simulink model "speedgoat_test_SN5659_R2021b_IO682"  (R2021b)
settings: Solver=FixedStepDiscrete  StartTime=0.0  StopTime=20  RelTol=1e-3
PreLoadFcn:
  | Ts_IO107 = 0.001;
  | Ts_IO107 = 0.001;
  | Ts_IO133 = 0.001
  | 
  | Ts_IO204 = 0.001;
  | 
  | 
  | Ts_IO503 = 0.01;
  | 
  | ts_IO612 = 1e-3;
  | Ts_IO682 = 0.005;
  | Ts_IO941 = 0.01;
InitFcn:
  | Ts_IO107 = 0.001;
  | Ts_IO107 = 0.001;
  | Ts_IO133 = 0.001
  | 
  | Ts_IO204 = 0.001;
  | 
  | 
  | Ts_IO503 = 0.01;
  | 
  | ts_IO612 = 1e-3;
  | Ts_IO682 = 0.005;
  | Ts_IO941 = 0.01;
StopFcn:
  | if isfile(['sdi_view_',bdroot,'.mldatx'])
  |  Simulink.sdi.clearPreferences();
  |  Simulink.sdi.view();
  |  pause(3);
  |  Simulink.sdi.loadView(['sdi_view_',bdroot,]);
  | end
undefined symbols (not defined in the file): IO682
libraries: speedgoatlib_IO682 x161, simulink x49
(part 1 of 3)
settings Model: Creator=yannick.orgas  LastModifiedBy=ACH
settings SolverCC: ConcurrentTasks=on  AlgebraicLoopSolver=TrustRegion  PositivePriorityOrder=on
settings DataIOCC: LimitDataPoints=on  SaveFormat=StructureWithTime
settings OptimizationCC: BlockReduction=off  OptimizeBlockIOStorage=off
settings DebuggingCC: TasksWithSamePriorityMsg=none  UnconnectedInputMsg=none  UnconnectedOutputMsg=none  UnconnectedLineMsg=none  SFMachineParentedDataDiag=warning
settings HardwareCC: ProdBitPerLong=64  ProdLongLongMode=on  ProdHWDeviceType=Intel->x86-64 (Linux 64)
settings RTWCC: Description=Simulink Real-Time  SystemTargetFile=slrealtime.tlc  TemplateMakefile=slrealtime_default_tmf  Toolchain=Simulink Real-Time Toolchain  BuildConfiguration=Faster Runs  CodeExecutionProfiling=on  TargetLang=C++
settings SimulinkRealTimeTargetCC: UseGCCFastMath=on

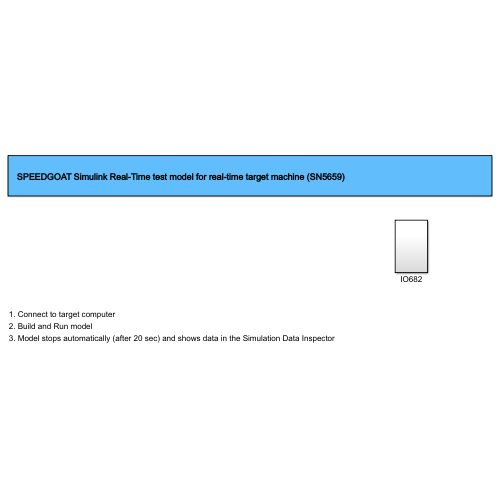
[thumbnail: Simulink's stored preview of the top-level diagram]
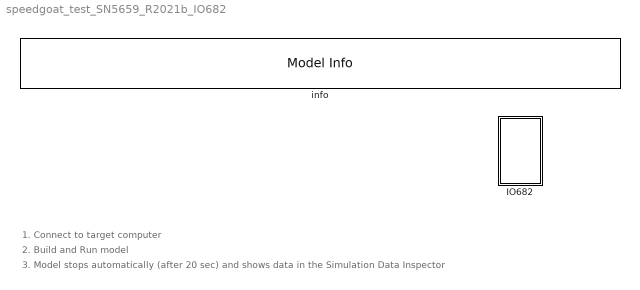
== system speedgoat_test_SN5659_R2021b_IO682 ==
  note: 1. Connect to target computer
  note: 2. Build and Run model
  note: 3. Model stops automatically (after 20 sec) and shows data in the Simulation Data Inspector
  IO682 : Subsystem
  info : simulink/Model-Wide Utilities/Model Info  Frame=on  DisplayStringWithTags=SPEEDGOAT Simulink Real-Time test model for real-time target machine (SN5659)  HorizontalTextAlignment=Left  LeftAlignmentValue=0.02

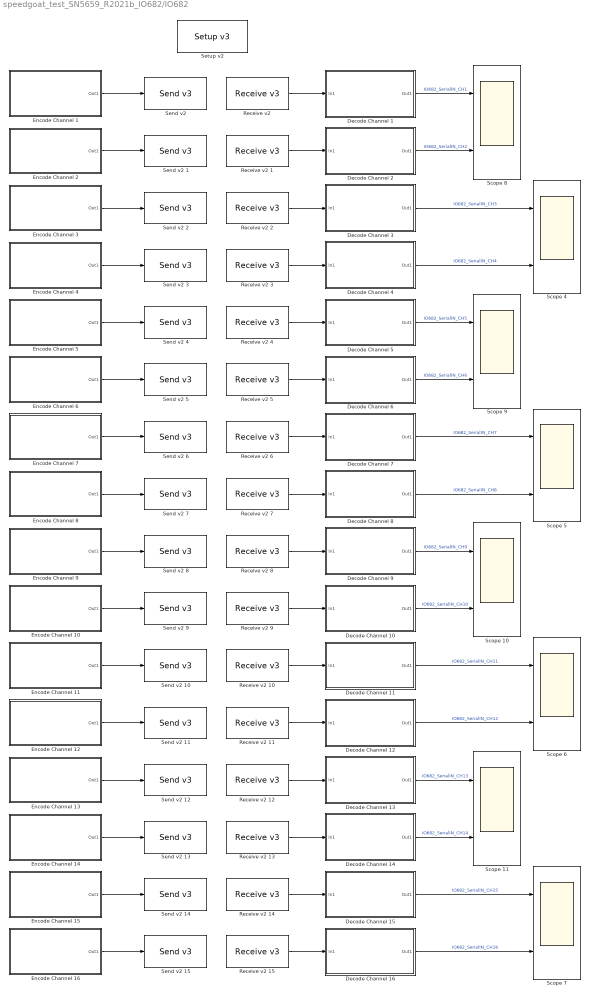
== system speedgoat_test_SN5659_R2021b_IO682/IO682 ==
  Decode Channel 1 : Subsystem
  Decode Channel 10 : Subsystem
  Decode Channel 11 : Subsystem
  Decode Channel 12 : Subsystem
  Decode Channel 13 : Subsystem
  Decode Channel 14 : Subsystem
  Decode Channel 15 : Subsystem
  Decode Channel 16 : Subsystem
  Decode Channel 2 : Subsystem
  Decode Channel 3 : Subsystem
  Decode Channel 4 : Subsystem
  Decode Channel 5 : Subsystem
  Decode Channel 6 : Subsystem
  Decode Channel 7 : Subsystem
  Decode Channel 8 : Subsystem
  Decode Channel 9 : Subsystem
  Encode Channel 1 : Subsystem
  Encode Channel 10 : Subsystem
  Encode Channel 11 : Subsystem
  Encode Channel 12 : Subsystem
  Encode Channel 13 : Subsystem
  Encode Channel 14 : Subsystem
  Encode Channel 15 : Subsystem
  Encode Channel 16 : Subsystem
  Encode Channel 2 : Subsystem
  Encode Channel 3 : Subsystem
  Encode Channel 4 : Subsystem
  Encode Channel 5 : Subsystem
  Encode Channel 6 : Subsystem
  Encode Channel 7 : Subsystem
  Encode Channel 8 : Subsystem
  Encode Channel 9 : Subsystem
  "Receive v2 " : speedgoatlib_IO682/Receive v3   parModuleId=1  parChannel=1  parMaxWords=50  parMinWords=1  parSampleTime=Ts_IO682
      settings: SourceProductName=Speedgoat I/O Blockset
  Receive v2 1 : speedgoatlib_IO682/Receive v3   parModuleId=1  parChannel=2  parMaxWords=50  parMinWords=1  parSampleTime=Ts_IO682
      settings: SourceProductName=Speedgoat I/O Blockset
  Receive v2 10 : speedgoatlib_IO682/Receive v3   parModuleId=1  parChannel=11  parMaxWords=50  parMinWords=1  parSampleTime=Ts_IO682
      settings: SourceProductName=Speedgoat I/O Blockset
  Receive v2 11 : speedgoatlib_IO682/Receive v3   parModuleId=1  parChannel=12  parMaxWords=50  parMinWords=1  parSampleTime=Ts_IO682
      settings: SourceProductName=Speedgoat I/O Blockset
  Receive v2 12 : speedgoatlib_IO682/Receive v3   parModuleId=1  parChannel=13  parMaxWords=50  parMinWords=1  parSampleTime=Ts_IO682
      settings: SourceProductName=Speedgoat I/O Blockset
  Receive v2 13 : speedgoatlib_IO682/Receive v3   parModuleId=1  parChannel=14  parMaxWords=50  parMinWords=1  parSampleTime=Ts_IO682
      settings: SourceProductName=Speedgoat I/O Blockset
  Receive v2 14 : speedgoatlib_IO682/Receive v3   parModuleId=1  parChannel=15  parMaxWords=50  parMinWords=1  parSampleTime=Ts_IO682
      settings: SourceProductName=Speedgoat I/O Blockset
  Receive v2 15 : speedgoatlib_IO682/Receive v3   parModuleId=1  parChannel=16  parMaxWords=50  parMinWords=1  parSampleTime=Ts_IO682
      settings: SourceProductName=Speedgoat I/O Blockset
  Receive v2 2 : speedgoatlib_IO682/Receive v3   parModuleId=1  parChannel=3  parMaxWords=50  parMinWords=1  parSampleTime=Ts_IO682
      settings: SourceProductName=Speedgoat I/O Blockset
  Receive v2 3 : speedgoatlib_IO682/Receive v3   parModuleId=1  parChannel=4  parMaxWords=50  parMinWords=1  parSampleTime=Ts_IO682
      settings: SourceProductName=Speedgoat I/O Blockset
  Receive v2 4 : speedgoatlib_IO682/Receive v3   parModuleId=1  parChannel=5  parMaxWords=50  parMinWords=1  parSampleTime=Ts_IO682
      settings: SourceProductName=Speedgoat I/O Blockset
  Receive v2 5 : speedgoatlib_IO682/Receive v3   parModuleId=1  parChannel=6  parMaxWords=50  parMinWords=1  parSampleTime=Ts_IO682
      settings: SourceProductName=Speedgoat I/O Blockset
  Receive v2 6 : speedgoatlib_IO682/Receive v3   parModuleId=1  parChannel=7  parMaxWords=50  parMinWords=1  parSampleTime=Ts_IO682
      settings: SourceProductName=Speedgoat I/O Blockset
  Receive v2 7 : speedgoatlib_IO682/Receive v3   parModuleId=1  parChannel=8  parMaxWords=50  parMinWords=1  parSampleTime=Ts_IO682
      settings: SourceProductName=Speedgoat I/O Blockset
  Receive v2 8 : speedgoatlib_IO682/Receive v3   parModuleId=1  parChannel=9  parMaxWords=50  parMinWords=1  parSampleTime=Ts_IO682
      settings: SourceProductName=Speedgoat I/O Blockset
  Receive v2 9 : speedgoatlib_IO682/Receive v3   parModuleId=1  parChannel=10  parMaxWords=50  parMinWords=1  parSampleTime=Ts_IO682
      settings: SourceProductName=Speedgoat I/O Blockset
  Scope {4..11} (8 alike) : Scope  NumInputPorts=2
  "Send v2 " : speedgoatlib_IO682/Send v3   parModuleId=1  parChannel=1  parSampleTime=Ts_IO682
      settings: SourceProductName=Speedgoat I/O Blockset
  Send v2 1 : speedgoatlib_IO682/Send v3   parModuleId=1  parChannel=2  parSampleTime=Ts_IO682
      settings: SourceProductName=Speedgoat I/O Blockset
  Send v2 10 : speedgoatlib_IO682/Send v3   parModuleId=1  parChannel=11  parSampleTime=Ts_IO682
      settings: SourceProductName=Speedgoat I/O Blockset
  Send v2 11 : speedgoatlib_IO682/Send v3   parModuleId=1  parChannel=12  parSampleTime=Ts_IO682
      settings: SourceProductName=Speedgoat I/O Blockset
  Send v2 12 : speedgoatlib_IO682/Send v3   parModuleId=1  parChannel=13  parSampleTime=Ts_IO682
      settings: SourceProductName=Speedgoat I/O Blockset
  Send v2 13 : speedgoatlib_IO682/Send v3   parModuleId=1  parChannel=14  parSampleTime=Ts_IO682
      settings: SourceProductName=Speedgoat I/O Blockset
  Send v2 14 : speedgoatlib_IO682/Send v3   parModuleId=1  parChannel=15  parSampleTime=Ts_IO682
      settings: SourceProductName=Speedgoat I/O Blockset
  Send v2 15 : speedgoatlib_IO682/Send v3   parModuleId=1  parChannel=16  parSampleTime=Ts_IO682
      settings: SourceProductName=Speedgoat I/O Blockset
  Send v2 2 : speedgoatlib_IO682/Send v3   parModuleId=1  parChannel=3  parSampleTime=Ts_IO682
      settings: SourceProductName=Speedgoat I/O Blockset
  Send v2 3 : speedgoatlib_IO682/Send v3   parModuleId=1  parChannel=4  parSampleTime=Ts_IO682
      settings: SourceProductName=Speedgoat I/O Blockset
  Send v2 4 : speedgoatlib_IO682/Send v3   parModuleId=1  parChannel=5  parSampleTime=Ts_IO682
      settings: SourceProductName=Speedgoat I/O Blockset
  Send v2 5 : speedgoatlib_IO682/Send v3   parModuleId=1  parChannel=6  parSampleTime=Ts_IO682
      settings: SourceProductName=Speedgoat I/O Blockset
  Send v2 6 : speedgoatlib_IO682/Send v3   parModuleId=1  parChannel=7  parSampleTime=Ts_IO682
      settings: SourceProductName=Speedgoat I/O Blockset
  Send v2 7 : speedgoatlib_IO682/Send v3   parModuleId=1  parChannel=8  parSampleTime=Ts_IO682
      settings: SourceProductName=Speedgoat I/O Blockset
  Send v2 8 : speedgoatlib_IO682/Send v3   parModuleId=1  parChannel=9  parSampleTime=Ts_IO682
      settings: SourceProductName=Speedgoat I/O Blockset
  Send v2 9 : speedgoatlib_IO682/Send v3   parModuleId=1  parChannel=10  parSampleTime=Ts_IO682
      settings: SourceProductName=Speedgoat I/O Blockset
  "Setup v2 " : speedgoatlib_IO682/Setup v3   parModuleId=1  parBoardVariant=IO682-16-16  parPciSlot=-1  parTimerCount=4000  parChannelMode=Manual  parInBitRate1=100000  parInBufferMode1=Individual  parInEnable1=on  parInParity1=on  parInInternalWrap1=off  parInBitRate2=100000  parInBufferMode2=Individual  parInEnable2=on  parInParity2=on  parInInternalWrap2=off  parInBitRate3=100000  parInBufferMode3=Individual  parInEnable3=on  parInParity3=on  parInInternalWrap3=off  parInBitRate4=100000  parInBufferMode4=Individual  parInEnable4=on  parInParity4=on  parInInternalWrap4=off  parInBitRate5=100000  parInBufferMode5=Individual  parInEnable5=on  parInParity5=on  parInInternalWrap5=off  parInBitRate6=100000  parInBufferMode6=Individual  parInEnable6=on  parInParity6=on  parInInternalWrap6=off  parInBitRate7=100000  parInBufferMode7=Individual  parInEnable7=on  parInParity7=on  parInInternalWrap7=off  parInBitRate8=100000  parInBufferMode8=Individual  parInEnable8=on  parInParity8=on  parInInternalWrap8=off  parInBitRate9=100000  parInBufferMode9=Individual  parInEnable9=on  parInParity9=on  parInInternalWrap9=off  parInBitRate10=100000  parInBufferMode10=Individual  parInEnable10=on  parInParity10=on  parInInternalWrap10=off  parInBitRate11=100000  parInBufferMode11=Individual  parInEnable11=on  parInParity11=on  parInInternalWrap11=off  parInBitRate12=100000  parInBufferMode12=Individual  parInEnable12=on  parInParity12=on  parInInternalWrap12=off  parInBitRate13=100000  parInBufferMode13=Individual  parInEnable13=on  parInParity13=on  parInInternalWrap13=off  parInBitRate14=100000  parInBufferMode14=Individual  parInEnable14=on  parInParity14=on  parInInternalWrap14=off  parInBitRate15=100000  parInBufferMode15=Individual  parInEnable15=on  parInParity15=on  parInInternalWrap15=off  parInBitRate16=100000  parInBufferMode16=Individual  parInEnable16=on  parInParity16=on  parInInternalWrap16=off  parOutBitRate1=100000  parOutParity1=Odd  parOutProtocolError1=None  parOutEnable1=on  parOutBitRate2=100000  parOutParity2=Odd  parOutProtocolError2=None  parOutEnable2=on  parOutBitRate3=100000  parOutParity3=Odd  parOutProtocolError3=None  parOutEnable3=on  parOutBitRate4=100000  parOutParity4=Odd  parOutProtocolError4=None  parOutEnable4=on  parOutBitRate5=100000  parOutParity5=Odd  parOutProtocolError5=None  parOutEnable5=on  parOutBitRate6=100000  parOutParity6=Odd  parOutProtocolError6=None  parOutEnable6=on  parOutBitRate7=100000  parOutParity7=Odd  parOutProtocolError7=None  parOutEnable7=on  parOutBitRate8=100000  parOutParity8=Odd  parOutProtocolError8=None  parOutEnable8=on  parOutBitRate9=100000  parOutParity9=Odd  parOutProtocolError9=None  parOutEnable9=on  parOutBitRate10=100000  parOutParity10=Odd  parOutProtocolError10=None  parOutEnable10=on  parOutBitRate11=100000  parOutParity11=Odd  parOutProtocolError11=None  parOutEnable11=on  parOutBitRate12=100000  parOutParity12=Odd  parOutProtocolError12=None  parOutEnable12=on  parOutBitRate13=100000  parOutParity13=Odd  parOutProtocolError13=None  parOutEnable13=on  parOutBitRate14=100000  parOutParity14=Odd  parOutProtocolError14=None  parOutEnable14=on  parOutBitRate15=100000  parOutParity15=Odd  parOutProtocolError15=None  parOutEnable15=on  parOutBitRate16=100000  parOutParity16=Odd  parOutProtocolError16=None  parOutEnable16=on  parChConfigFile=''  parScheduleMode=Manual  parScheduledMsgConfigFile=''  parHwDeviceId=hex2dec('0830')  parTimeSource=Internal timer  parChInConfig=[158 8 7 7 1;158 8 7 7 1;158 8 7 7 1;158 8 7 7 1;158 8 7 7 1;158 8 7 7 1;158 8 7 7 1;158 8 7 7 1;158 8 7 7 1;158 8 7 7 1;158 8 7 7 1;158 8 7 7 1;158 8 7 7 1;158 8 7 7 1;158 8 7 7 1;158 8 7 7 1]  parChOutConfig=[158 0 4 7;158 0 4 7;158 0 4 7;158 0 4 7;158 0 4 7;158 0 4 7;158 0 4 7;158 0 4 7;158 0 4 7;158 0 4 7;158 0 4 7;158 0 4 7;158 0 4 7;158 0 4 7;158 0 4 7;158 0 4 7]  parScheduledMessages=0
      settings: SourceProductName=Speedgoat I/O Blockset
  wires:
  Receive v2 3/1 -> Decode Channel 4/1(In1)
  Decode Channel 15/1(Out1) -> Scope 7/1  "IO682_SerialIN_CH15"
  "Receive v2 "/1 -> Decode Channel 1/1(In1)
  Receive v2 13/1 -> Decode Channel 14/1(In1)
  Decode Channel 11/1(Out1) -> Scope 6/1  "IO682_SerialIN_CH11"
  Encode Channel 15/1(Out1) -> Send v2 14/1
  Receive v2 8/1 -> Decode Channel 9/1(In1)
  Decode Channel 16/1(Out1) -> Scope 7/2  "IO682_SerialIN_CH16"
  Receive v2 15/1 -> Decode Channel 16/1(In1)
  Encode Channel 13/1(Out1) -> Send v2 12/1
  Encode Channel 14/1(Out1) -> Send v2 13/1
  Decode Channel 12/1(Out1) -> Scope 6/2  "IO682_SerialIN_CH12"
  Decode Channel 3/1(Out1) -> Scope 4/1  "IO682_SerialIN_CH3"
  Receive v2 14/1 -> Decode Channel 15/1(In1)
  Encode Channel 1/1(Out1) -> "Send v2 "/1
  Decode Channel 5/1(Out1) -> Scope 9/1  "IO682_SerialIN_CH5"
  Encode Channel 7/1(Out1) -> Send v2 6/1
  Receive v2 7/1 -> Decode Channel 8/1(In1)
  Decode Channel 14/1(Out1) -> Scope 11/2  "IO682_SerialIN_CH14"
  Decode Channel 10/1(Out1) -> Scope 10/2  "IO682_SerialIN_CH10"
  Encode Channel 9/1(Out1) -> Send v2 8/1
  Receive v2 2/1 -> Decode Channel 3/1(In1)
  Receive v2 10/1 -> Decode Channel 11/1(In1)
  Decode Channel 8/1(Out1) -> Scope 5/2  "IO682_SerialIN_CH8"
  Encode Channel 4/1(Out1) -> Send v2 3/1
  Encode Channel 6/1(Out1) -> Send v2 5/1
  Encode Channel 2/1(Out1) -> Send v2 1/1
  Receive v2 9/1 -> Decode Channel 10/1(In1)
  Encode Channel 16/1(Out1) -> Send v2 15/1
  Decode Channel 9/1(Out1) -> Scope 10/1  "IO682_SerialIN_CH9"
  Receive v2 11/1 -> Decode Channel 12/1(In1)
  Encode Channel 11/1(Out1) -> Send v2 10/1
  Encode Channel 10/1(Out1) -> Send v2 9/1
  Receive v2 12/1 -> Decode Channel 13/1(In1)
  Decode Channel 1/1(Out1) -> Scope 8/1  "IO682_SerialIN_CH1"
  Decode Channel 2/1(Out1) -> Scope 8/2  "IO682_SerialIN_CH2"
  Decode Channel 13/1(Out1) -> Scope 11/1  "IO682_SerialIN_CH13"
  Decode Channel 6/1(Out1) -> Scope 9/2  "IO682_SerialIN_CH6"
  Receive v2 1/1 -> Decode Channel 2/1(In1)
  Encode Channel 8/1(Out1) -> Send v2 7/1
  Receive v2 5/1 -> Decode Channel 6/1(In1)
  Receive v2 4/1 -> Decode Channel 5/1(In1)
  Decode Channel 7/1(Out1) -> Scope 5/1  "IO682_SerialIN_CH7"
  Encode Channel 5/1(Out1) -> Send v2 4/1
  Receive v2 6/1 -> Decode Channel 7/1(In1)
  Decode Channel 4/1(Out1) -> Scope 4/2  "IO682_SerialIN_CH4"
  Encode Channel 3/1(Out1) -> Send v2 2/1
  Encode Channel 12/1(Out1) -> Send v2 11/1

== system speedgoat_test_SN5659_R2021b_IO682/IO682/Decode Channel 1 ==
  note: Because of the limited number of bits
      | that are encoded and sent by ARINC,
      | these values may differ from values
      | on the input side.
  In1 : Inport
  Decode 1 : speedgoatlib_IO682/Decode v2   parMode=Standard  parLabel=100  parDataType=[1]  parResolution=[1024]  parSyncMask=hex2dec('0x0')  parSyncValue=hex2dec('0x0')  parCustomDataType=Raw  parDataLSB=9  parDataMSB=31  parBitPosition=[9, 31]  parScaleBNR=1  parExponent=8  parMantissa=14  parTimeTags=off  parHoldLastVal=on  parStatus=off
      settings: SourceProductName=Simulink Real-Time: Speedgoat I/O Blockset
  Decode 3 : speedgoatlib_IO682/Decode v2   parMode=Standard  parLabel=102  parDataType=[1]  parResolution=[65536]  parSyncMask=hex2dec('0x0')  parSyncValue=hex2dec('0x0')  parCustomDataType=Raw  parDataLSB=9  parDataMSB=31  parBitPosition=[9, 31]  parScaleBNR=1  parExponent=8  parMantissa=14  parTimeTags=off  parHoldLastVal=on  parStatus=off
      settings: SourceProductName=Simulink Real-Time: Speedgoat I/O Blockset
  Decode 4 : speedgoatlib_IO682/Decode v2   parMode=Standard  parLabel=103  parDataType=[1]  parResolution=[1024]  parSyncMask=hex2dec('0x0')  parSyncValue=hex2dec('0x0')  parCustomDataType=Raw  parDataLSB=9  parDataMSB=31  parBitPosition=[9, 31]  parScaleBNR=1  parExponent=8  parMantissa=14  parTimeTags=off  parHoldLastVal=on  parStatus=off
      settings: SourceProductName=Simulink Real-Time: Speedgoat I/O Blockset
  Decode 5 : speedgoatlib_IO682/Decode v2   parMode=Standard  parLabel=101  parDataType=[2]  parResolution=[.1]  parSyncMask=hex2dec('0x0')  parSyncValue=hex2dec('0x0')  parCustomDataType=Raw  parDataLSB=9  parDataMSB=31  parBitPosition=[9, 31]  parScaleBNR=1  parExponent=8  parMantissa=14  parTimeTags=off  parHoldLastVal=on  parStatus=off
      settings: SourceProductName=Simulink Real-Time: Speedgoat I/O Blockset
  Mux : Mux
  Out1 : Outport
  wires:
  In1/1 -> Decode 3/1, Decode 4/1, Decode 5/1, Decode 1/1
  Mux/1 -> Out1/1
  Decode 5/1 -> Mux/2
  Decode 1/1 -> Mux/1
  Decode 3/1 -> Mux/3
  Decode 4/1 -> Mux/4

== system speedgoat_test_SN5659_R2021b_IO682/IO682/Decode Channel 10 ==
  In1 : Inport
  Decode 1 : speedgoatlib_IO682/Decode v2   parMode=Standard  parLabel=100  parDataType=[1]  parResolution=[1024]  parSyncMask=hex2dec('0x0')  parSyncValue=hex2dec('0x0')  parCustomDataType=Raw  parDataLSB=9  parDataMSB=31  parBitPosition=[9, 31]  parScaleBNR=1  parExponent=8  parMantissa=14  parTimeTags=off  parHoldLastVal=on  parStatus=off
      settings: SourceProductName=Simulink Real-Time: Speedgoat I/O Blockset
  Decode 2 : speedgoatlib_IO682/Decode v2   parMode=Standard  parLabel=101  parDataType=[2]  parResolution=[.1]  parSyncMask=hex2dec('0x0')  parSyncValue=hex2dec('0x0')  parCustomDataType=Raw  parDataLSB=9  parDataMSB=31  parBitPosition=[9, 31]  parScaleBNR=1  parExponent=8  parMantissa=14  parTimeTags=off  parHoldLastVal=on  parStatus=off
      settings: SourceProductName=Simulink Real-Time: Speedgoat I/O Blockset
  Decode 3 : speedgoatlib_IO682/Decode v2   parMode=Standard  parLabel=102  parDataType=[1]  parResolution=[65536]  parSyncMask=hex2dec('0x0')  parSyncValue=hex2dec('0x0')  parCustomDataType=Raw  parDataLSB=9  parDataMSB=31  parBitPosition=[9, 31]  parScaleBNR=1  parExponent=8  parMantissa=14  parTimeTags=off  parHoldLastVal=on  parStatus=off
      settings: SourceProductName=Simulink Real-Time: Speedgoat I/O Blockset
  Decode 4 : speedgoatlib_IO682/Decode v2   parMode=Standard  parLabel=103  parDataType=[1]  parResolution=[1024]  parSyncMask=hex2dec('0x0')  parSyncValue=hex2dec('0x0')  parCustomDataType=Raw  parDataLSB=9  parDataMSB=31  parBitPosition=[9, 31]  parScaleBNR=1  parExponent=8  parMantissa=14  parTimeTags=off  parHoldLastVal=on  parStatus=off
      settings: SourceProductName=Simulink Real-Time: Speedgoat I/O Blockset
  Mux : Mux
  Out1 : Outport
  wires:
  Decode 1/1 -> Mux/1
  In1/1 -> Decode 4/1, Decode 3/1, Decode 2/1, Decode 1/1
  Mux/1 -> Out1/1
  Decode 4/1 -> Mux/4
  Decode 3/1 -> Mux/3
  Decode 2/1 -> Mux/2

== system speedgoat_test_SN5659_R2021b_IO682/IO682/Decode Channel 11 ==
  In1 : Inport
  Decode 1 : speedgoatlib_IO682/Decode v2   parMode=Standard  parLabel=100  parDataType=[1]  parResolution=[1024]  parSyncMask=hex2dec('0x0')  parSyncValue=hex2dec('0x0')  parCustomDataType=Raw  parDataLSB=9  parDataMSB=31  parBitPosition=[9, 31]  parScaleBNR=1  parExponent=8  parMantissa=14  parTimeTags=off  parHoldLastVal=on  parStatus=off
      settings: SourceProductName=Simulink Real-Time: Speedgoat I/O Blockset
  Decode 2 : speedgoatlib_IO682/Decode v2   parMode=Standard  parLabel=101  parDataType=[2]  parResolution=[.1]  parSyncMask=hex2dec('0x0')  parSyncValue=hex2dec('0x0')  parCustomDataType=Raw  parDataLSB=9  parDataMSB=31  parBitPosition=[9, 31]  parScaleBNR=1  parExponent=8  parMantissa=14  parTimeTags=off  parHoldLastVal=on  parStatus=off
      settings: SourceProductName=Simulink Real-Time: Speedgoat I/O Blockset
  Decode 3 : speedgoatlib_IO682/Decode v2   parMode=Standard  parLabel=102  parDataType=[1]  parResolution=[65536]  parSyncMask=hex2dec('0x0')  parSyncValue=hex2dec('0x0')  parCustomDataType=Raw  parDataLSB=9  parDataMSB=31  parBitPosition=[9, 31]  parScaleBNR=1  parExponent=8  parMantissa=14  parTimeTags=off  parHoldLastVal=on  parStatus=off
      settings: SourceProductName=Simulink Real-Time: Speedgoat I/O Blockset
  Decode 4 : speedgoatlib_IO682/Decode v2   parMode=Standard  parLabel=103  parDataType=[1]  parResolution=[1024]  parSyncMask=hex2dec('0x0')  parSyncValue=hex2dec('0x0')  parCustomDataType=Raw  parDataLSB=9  parDataMSB=31  parBitPosition=[9, 31]  parScaleBNR=1  parExponent=8  parMantissa=14  parTimeTags=off  parHoldLastVal=on  parStatus=off
      settings: SourceProductName=Simulink Real-Time: Speedgoat I/O Blockset
  Mux : Mux
  Out1 : Outport
  wires:
  Decode 1/1 -> Mux/1
  Decode 2/1 -> Mux/2
  Decode 4/1 -> Mux/4
  Decode 3/1 -> Mux/3
  Mux/1 -> Out1/1
  In1/1 -> Decode 4/1, Decode 3/1, Decode 2/1, Decode 1/1

== system speedgoat_test_SN5659_R2021b_IO682/IO682/Decode Channel 12 ==
  In1 : Inport
  Decode 1 : speedgoatlib_IO682/Decode v2   parMode=Standard  parLabel=100  parDataType=[1]  parResolution=[1024]  parSyncMask=hex2dec('0x0')  parSyncValue=hex2dec('0x0')  parCustomDataType=Raw  parDataLSB=9  parDataMSB=31  parBitPosition=[9, 31]  parScaleBNR=1  parExponent=8  parMantissa=14  parTimeTags=off  parHoldLastVal=on  parStatus=off
      settings: SourceProductName=Simulink Real-Time: Speedgoat I/O Blockset
  Decode 2 : speedgoatlib_IO682/Decode v2   parMode=Standard  parLabel=101  parDataType=[2]  parResolution=[.1]  parSyncMask=hex2dec('0x0')  parSyncValue=hex2dec('0x0')  parCustomDataType=Raw  parDataLSB=9  parDataMSB=31  parBitPosition=[9, 31]  parScaleBNR=1  parExponent=8  parMantissa=14  parTimeTags=off  parHoldLastVal=on  parStatus=off
      settings: SourceProductName=Simulink Real-Time: Speedgoat I/O Blockset
  Decode 3 : speedgoatlib_IO682/Decode v2   parMode=Standard  parLabel=102  parDataType=[1]  parResolution=[65536]  parSyncMask=hex2dec('0x0')  parSyncValue=hex2dec('0x0')  parCustomDataType=Raw  parDataLSB=9  parDataMSB=31  parBitPosition=[9, 31]  parScaleBNR=1  parExponent=8  parMantissa=14  parTimeTags=off  parHoldLastVal=on  parStatus=off
      settings: SourceProductName=Simulink Real-Time: Speedgoat I/O Blockset
  Decode 4 : speedgoatlib_IO682/Decode v2   parMode=Standard  parLabel=103  parDataType=[1]  parResolution=[1024]  parSyncMask=hex2dec('0x0')  parSyncValue=hex2dec('0x0')  parCustomDataType=Raw  parDataLSB=9  parDataMSB=31  parBitPosition=[9, 31]  parScaleBNR=1  parExponent=8  parMantissa=14  parTimeTags=off  parHoldLastVal=on  parStatus=off
      settings: SourceProductName=Simulink Real-Time: Speedgoat I/O Blockset
  Mux : Mux
  Out1 : Outport
  wires:
  Decode 1/1 -> Mux/1
  Decode 2/1 -> Mux/2
  Decode 4/1 -> Mux/4
  Decode 3/1 -> Mux/3
  Mux/1 -> Out1/1
  In1/1 -> Decode 4/1, Decode 3/1, Decode 2/1, Decode 1/1

== system speedgoat_test_SN5659_R2021b_IO682/IO682/Decode Channel 13 ==
  note: Because of the limited number of bits
      | that are encoded and sent by ARINC,
      | these values may differ from values
      | on the input side.
  In1 : Inport
  Decode 1 : speedgoatlib_IO682/Decode v2   parMode=Standard  parLabel=100  parDataType=[1]  parResolution=[1024]  parSyncMask=hex2dec('0x0')  parSyncValue=hex2dec('0x0')  parCustomDataType=Raw  parDataLSB=9  parDataMSB=31  parBitPosition=[9, 31]  parScaleBNR=1  parExponent=8  parMantissa=14  parTimeTags=off  parHoldLastVal=on  parStatus=off
      settings: SourceProductName=Simulink Real-Time: Speedgoat I/O Blockset
  Decode 3 : speedgoatlib_IO682/Decode v2   parMode=Standard  parLabel=102  parDataType=[1]  parResolution=[65536]  parSyncMask=hex2dec('0x0')  parSyncValue=hex2dec('0x0')  parCustomDataType=Raw  parDataLSB=9  parDataMSB=31  parBitPosition=[9, 31]  parScaleBNR=1  parExponent=8  parMantissa=14  parTimeTags=off  parHoldLastVal=on  parStatus=off
      settings: SourceProductName=Simulink Real-Time: Speedgoat I/O Blockset
  Decode 4 : speedgoatlib_IO682/Decode v2   parMode=Standard  parLabel=103  parDataType=[1]  parResolution=[1024]  parSyncMask=hex2dec('0x0')  parSyncValue=hex2dec('0x0')  parCustomDataType=Raw  parDataLSB=9  parDataMSB=31  parBitPosition=[9, 31]  parScaleBNR=1  parExponent=8  parMantissa=14  parTimeTags=off  parHoldLastVal=on  parStatus=off
      settings: SourceProductName=Simulink Real-Time: Speedgoat I/O Blockset
  Decode 5 : speedgoatlib_IO682/Decode v2   parMode=Standard  parLabel=101  parDataType=[2]  parResolution=[.1]  parSyncMask=hex2dec('0x0')  parSyncValue=hex2dec('0x0')  parCustomDataType=Raw  parDataLSB=9  parDataMSB=31  parBitPosition=[9, 31]  parScaleBNR=1  parExponent=8  parMantissa=14  parTimeTags=off  parHoldLastVal=on  parStatus=off
      settings: SourceProductName=Simulink Real-Time: Speedgoat I/O Blockset
  Mux : Mux
  Out1 : Outport
  wires:
  In1/1 -> Decode 3/1, Decode 4/1, Decode 5/1, Decode 1/1
  Mux/1 -> Out1/1
  Decode 5/1 -> Mux/2
  Decode 1/1 -> Mux/1
  Decode 3/1 -> Mux/3
  Decode 4/1 -> Mux/4

== system speedgoat_test_SN5659_R2021b_IO682/IO682/Decode Channel 14 ==
  In1 : Inport
  Decode 1 : speedgoatlib_IO682/Decode v2   parMode=Standard  parLabel=100  parDataType=[1]  parResolution=[1024]  parSyncMask=hex2dec('0x0')  parSyncValue=hex2dec('0x0')  parCustomDataType=Raw  parDataLSB=9  parDataMSB=31  parBitPosition=[9, 31]  parScaleBNR=1  parExponent=8  parMantissa=14  parTimeTags=off  parHoldLastVal=on  parStatus=off
      settings: SourceProductName=Simulink Real-Time: Speedgoat I/O Blockset
  Decode 2 : speedgoatlib_IO682/Decode v2   parMode=Standard  parLabel=101  parDataType=[2]  parResolution=[.1]  parSyncMask=hex2dec('0x0')  parSyncValue=hex2dec('0x0')  parCustomDataType=Raw  parDataLSB=9  parDataMSB=31  parBitPosition=[9, 31]  parScaleBNR=1  parExponent=8  parMantissa=14  parTimeTags=off  parHoldLastVal=on  parStatus=off
      settings: SourceProductName=Simulink Real-Time: Speedgoat I/O Blockset
  Decode 3 : speedgoatlib_IO682/Decode v2   parMode=Standard  parLabel=102  parDataType=[1]  parResolution=[65536]  parSyncMask=hex2dec('0x0')  parSyncValue=hex2dec('0x0')  parCustomDataType=Raw  parDataLSB=9  parDataMSB=31  parBitPosition=[9, 31]  parScaleBNR=1  parExponent=8  parMantissa=14  parTimeTags=off  parHoldLastVal=on  parStatus=off
      settings: SourceProductName=Simulink Real-Time: Speedgoat I/O Blockset
  Decode 4 : speedgoatlib_IO682/Decode v2   parMode=Standard  parLabel=103  parDataType=[1]  parResolution=[1024]  parSyncMask=hex2dec('0x0')  parSyncValue=hex2dec('0x0')  parCustomDataType=Raw  parDataLSB=9  parDataMSB=31  parBitPosition=[9, 31]  parScaleBNR=1  parExponent=8  parMantissa=14  parTimeTags=off  parHoldLastVal=on  parStatus=off
      settings: SourceProductName=Simulink Real-Time: Speedgoat I/O Blockset
  Mux : Mux
  Out1 : Outport
  wires:
  Decode 1/1 -> Mux/1
  In1/1 -> Decode 4/1, Decode 3/1, Decode 2/1, Decode 1/1
  Mux/1 -> Out1/1
  Decode 4/1 -> Mux/4
  Decode 3/1 -> Mux/3
  Decode 2/1 -> Mux/2

== system speedgoat_test_SN5659_R2021b_IO682/IO682/Decode Channel 15 ==
  In1 : Inport
  Decode 1 : speedgoatlib_IO682/Decode v2   parMode=Standard  parLabel=100  parDataType=[1]  parResolution=[1024]  parSyncMask=hex2dec('0x0')  parSyncValue=hex2dec('0x0')  parCustomDataType=Raw  parDataLSB=9  parDataMSB=31  parBitPosition=[9, 31]  parScaleBNR=1  parExponent=8  parMantissa=14  parTimeTags=off  parHoldLastVal=on  parStatus=off
      settings: SourceProductName=Simulink Real-Time: Speedgoat I/O Blockset
  Decode 2 : speedgoatlib_IO682/Decode v2   parMode=Standard  parLabel=101  parDataType=[2]  parResolution=[.1]  parSyncMask=hex2dec('0x0')  parSyncValue=hex2dec('0x0')  parCustomDataType=Raw  parDataLSB=9  parDataMSB=31  parBitPosition=[9, 31]  parScaleBNR=1  parExponent=8  parMantissa=14  parTimeTags=off  parHoldLastVal=on  parStatus=off
      settings: SourceProductName=Simulink Real-Time: Speedgoat I/O Blockset
  Decode 3 : speedgoatlib_IO682/Decode v2   parMode=Standard  parLabel=102  parDataType=[1]  parResolution=[65536]  parSyncMask=hex2dec('0x0')  parSyncValue=hex2dec('0x0')  parCustomDataType=Raw  parDataLSB=9  parDataMSB=31  parBitPosition=[9, 31]  parScaleBNR=1  parExponent=8  parMantissa=14  parTimeTags=off  parHoldLastVal=on  parStatus=off
      settings: SourceProductName=Simulink Real-Time: Speedgoat I/O Blockset
  Decode 4 : speedgoatlib_IO682/Decode v2   parMode=Standard  parLabel=103  parDataType=[1]  parResolution=[1024]  parSyncMask=hex2dec('0x0')  parSyncValue=hex2dec('0x0')  parCustomDataType=Raw  parDataLSB=9  parDataMSB=31  parBitPosition=[9, 31]  parScaleBNR=1  parExponent=8  parMantissa=14  parTimeTags=off  parHoldLastVal=on  parStatus=off
      settings: SourceProductName=Simulink Real-Time: Speedgoat I/O Blockset
  Mux : Mux
  Out1 : Outport
  wires:
  Decode 1/1 -> Mux/1
  Decode 2/1 -> Mux/2
  Decode 4/1 -> Mux/4
  Decode 3/1 -> Mux/3
  Mux/1 -> Out1/1
  In1/1 -> Decode 4/1, Decode 3/1, Decode 2/1, Decode 1/1

== system speedgoat_test_SN5659_R2021b_IO682/IO682/Decode Channel 16 ==
  In1 : Inport
  Decode 1 : speedgoatlib_IO682/Decode v2   parMode=Standard  parLabel=100  parDataType=[1]  parResolution=[1024]  parSyncMask=hex2dec('0x0')  parSyncValue=hex2dec('0x0')  parCustomDataType=Raw  parDataLSB=9  parDataMSB=31  parBitPosition=[9, 31]  parScaleBNR=1  parExponent=8  parMantissa=14  parTimeTags=off  parHoldLastVal=on  parStatus=off
      settings: SourceProductName=Simulink Real-Time: Speedgoat I/O Blockset
  Decode 2 : speedgoatlib_IO682/Decode v2   parMode=Standard  parLabel=101  parDataType=[2]  parResolution=[.1]  parSyncMask=hex2dec('0x0')  parSyncValue=hex2dec('0x0')  parCustomDataType=Raw  parDataLSB=9  parDataMSB=31  parBitPosition=[9, 31]  parScaleBNR=1  parExponent=8  parMantissa=14  parTimeTags=off  parHoldLastVal=on  parStatus=off
      settings: SourceProductName=Simulink Real-Time: Speedgoat I/O Blockset
  Decode 3 : speedgoatlib_IO682/Decode v2   parMode=Standard  parLabel=102  parDataType=[1]  parResolution=[65536]  parSyncMask=hex2dec('0x0')  parSyncValue=hex2dec('0x0')  parCustomDataType=Raw  parDataLSB=9  parDataMSB=31  parBitPosition=[9, 31]  parScaleBNR=1  parExponent=8  parMantissa=14  parTimeTags=off  parHoldLastVal=on  parStatus=off
      settings: SourceProductName=Simulink Real-Time: Speedgoat I/O Blockset
  Decode 4 : speedgoatlib_IO682/Decode v2   parMode=Standard  parLabel=103  parDataType=[1]  parResolution=[1024]  parSyncMask=hex2dec('0x0')  parSyncValue=hex2dec('0x0')  parCustomDataType=Raw  parDataLSB=9  parDataMSB=31  parBitPosition=[9, 31]  parScaleBNR=1  parExponent=8  parMantissa=14  parTimeTags=off  parHoldLastVal=on  parStatus=off
      settings: SourceProductName=Simulink Real-Time: Speedgoat I/O Blockset
  Mux : Mux
  Out1 : Outport
  wires:
  Decode 1/1 -> Mux/1
  Decode 2/1 -> Mux/2
  Decode 4/1 -> Mux/4
  Decode 3/1 -> Mux/3
  Mux/1 -> Out1/1
  In1/1 -> Decode 4/1, Decode 3/1, Decode 2/1, Decode 1/1

== system speedgoat_test_SN5659_R2021b_IO682/IO682/Decode Channel 2 ==
  In1 : Inport
  Decode 1 : speedgoatlib_IO682/Decode v2   parMode=Standard  parLabel=100  parDataType=[1]  parResolution=[1024]  parSyncMask=hex2dec('0x0')  parSyncValue=hex2dec('0x0')  parCustomDataType=Raw  parDataLSB=9  parDataMSB=31  parBitPosition=[9, 31]  parScaleBNR=1  parExponent=8  parMantissa=14  parTimeTags=off  parHoldLastVal=on  parStatus=off
      settings: SourceProductName=Simulink Real-Time: Speedgoat I/O Blockset
  Decode 2 : speedgoatlib_IO682/Decode v2   parMode=Standard  parLabel=101  parDataType=[2]  parResolution=[.1]  parSyncMask=hex2dec('0x0')  parSyncValue=hex2dec('0x0')  parCustomDataType=Raw  parDataLSB=9  parDataMSB=31  parBitPosition=[9, 31]  parScaleBNR=1  parExponent=8  parMantissa=14  parTimeTags=off  parHoldLastVal=on  parStatus=off
      settings: SourceProductName=Simulink Real-Time: Speedgoat I/O Blockset
  Decode 3 : speedgoatlib_IO682/Decode v2   parMode=Standard  parLabel=102  parDataType=[1]  parResolution=[65536]  parSyncMask=hex2dec('0x0')  parSyncValue=hex2dec('0x0')  parCustomDataType=Raw  parDataLSB=9  parDataMSB=31  parBitPosition=[9, 31]  parScaleBNR=1  parExponent=8  parMantissa=14  parTimeTags=off  parHoldLastVal=on  parStatus=off
      settings: SourceProductName=Simulink Real-Time: Speedgoat I/O Blockset
  Decode 4 : speedgoatlib_IO682/Decode v2   parMode=Standard  parLabel=103  parDataType=[1]  parResolution=[1024]  parSyncMask=hex2dec('0x0')  parSyncValue=hex2dec('0x0')  parCustomDataType=Raw  parDataLSB=9  parDataMSB=31  parBitPosition=[9, 31]  parScaleBNR=1  parExponent=8  parMantissa=14  parTimeTags=off  parHoldLastVal=on  parStatus=off
      settings: SourceProductName=Simulink Real-Time: Speedgoat I/O Blockset
  Mux : Mux
  Out1 : Outport
  wires:
  Decode 1/1 -> Mux/1
  In1/1 -> Decode 4/1, Decode 3/1, Decode 2/1, Decode 1/1
  Mux/1 -> Out1/1
  Decode 4/1 -> Mux/4
  Decode 3/1 -> Mux/3
  Decode 2/1 -> Mux/2

== system speedgoat_test_SN5659_R2021b_IO682/IO682/Decode Channel 3 ==
  In1 : Inport
  Decode 1 : speedgoatlib_IO682/Decode v2   parMode=Standard  parLabel=100  parDataType=[1]  parResolution=[1024]  parSyncMask=hex2dec('0x0')  parSyncValue=hex2dec('0x0')  parCustomDataType=Raw  parDataLSB=9  parDataMSB=31  parBitPosition=[9, 31]  parScaleBNR=1  parExponent=8  parMantissa=14  parTimeTags=off  parHoldLastVal=on  parStatus=off
      settings: SourceProductName=Simulink Real-Time: Speedgoat I/O Blockset
  Decode 2 : speedgoatlib_IO682/Decode v2   parMode=Standard  parLabel=101  parDataType=[2]  parResolution=[.1]  parSyncMask=hex2dec('0x0')  parSyncValue=hex2dec('0x0')  parCustomDataType=Raw  parDataLSB=9  parDataMSB=31  parBitPosition=[9, 31]  parScaleBNR=1  parExponent=8  parMantissa=14  parTimeTags=off  parHoldLastVal=on  parStatus=off
      settings: SourceProductName=Simulink Real-Time: Speedgoat I/O Blockset
  Decode 3 : speedgoatlib_IO682/Decode v2   parMode=Standard  parLabel=102  parDataType=[1]  parResolution=[65536]  parSyncMask=hex2dec('0x0')  parSyncValue=hex2dec('0x0')  parCustomDataType=Raw  parDataLSB=9  parDataMSB=31  parBitPosition=[9, 31]  parScaleBNR=1  parExponent=8  parMantissa=14  parTimeTags=off  parHoldLastVal=on  parStatus=off
      settings: SourceProductName=Simulink Real-Time: Speedgoat I/O Blockset
  Decode 4 : speedgoatlib_IO682/Decode v2   parMode=Standard  parLabel=103  parDataType=[1]  parResolution=[1024]  parSyncMask=hex2dec('0x0')  parSyncValue=hex2dec('0x0')  parCustomDataType=Raw  parDataLSB=9  parDataMSB=31  parBitPosition=[9, 31]  parScaleBNR=1  parExponent=8  parMantissa=14  parTimeTags=off  parHoldLastVal=on  parStatus=off
      settings: SourceProductName=Simulink Real-Time: Speedgoat I/O Blockset
  Mux : Mux
  Out1 : Outport
  wires:
  Decode 1/1 -> Mux/1
  Decode 2/1 -> Mux/2
  Decode 4/1 -> Mux/4
  Decode 3/1 -> Mux/3
  Mux/1 -> Out1/1
  In1/1 -> Decode 4/1, Decode 3/1, Decode 2/1, Decode 1/1

== system speedgoat_test_SN5659_R2021b_IO682/IO682/Decode Channel 4 ==
  In1 : Inport
  Decode 1 : speedgoatlib_IO682/Decode v2   parMode=Standard  parLabel=100  parDataType=[1]  parResolution=[1024]  parSyncMask=hex2dec('0x0')  parSyncValue=hex2dec('0x0')  parCustomDataType=Raw  parDataLSB=9  parDataMSB=31  parBitPosition=[9, 31]  parScaleBNR=1  parExponent=8  parMantissa=14  parTimeTags=off  parHoldLastVal=on  parStatus=off
      settings: SourceProductName=Simulink Real-Time: Speedgoat I/O Blockset
  Decode 2 : speedgoatlib_IO682/Decode v2   parMode=Standard  parLabel=101  parDataType=[2]  parResolution=[.1]  parSyncMask=hex2dec('0x0')  parSyncValue=hex2dec('0x0')  parCustomDataType=Raw  parDataLSB=9  parDataMSB=31  parBitPosition=[9, 31]  parScaleBNR=1  parExponent=8  parMantissa=14  parTimeTags=off  parHoldLastVal=on  parStatus=off
      settings: SourceProductName=Simulink Real-Time: Speedgoat I/O Blockset
  Decode 3 : speedgoatlib_IO682/Decode v2   parMode=Standard  parLabel=102  parDataType=[1]  parResolution=[65536]  parSyncMask=hex2dec('0x0')  parSyncValue=hex2dec('0x0')  parCustomDataType=Raw  parDataLSB=9  parDataMSB=31  parBitPosition=[9, 31]  parScaleBNR=1  parExponent=8  parMantissa=14  parTimeTags=off  parHoldLastVal=on  parStatus=off
      settings: SourceProductName=Simulink Real-Time: Speedgoat I/O Blockset
  Decode 4 : speedgoatlib_IO682/Decode v2   parMode=Standard  parLabel=103  parDataType=[1]  parResolution=[1024]  parSyncMask=hex2dec('0x0')  parSyncValue=hex2dec('0x0')  parCustomDataType=Raw  parDataLSB=9  parDataMSB=31  parBitPosition=[9, 31]  parScaleBNR=1  parExponent=8  parMantissa=14  parTimeTags=off  parHoldLastVal=on  parStatus=off
      settings: SourceProductName=Simulink Real-Time: Speedgoat I/O Blockset
  Mux : Mux
  Out1 : Outport
  wires:
  Decode 1/1 -> Mux/1
  Decode 2/1 -> Mux/2
  Decode 4/1 -> Mux/4
  Decode 3/1 -> Mux/3
  Mux/1 -> Out1/1
  In1/1 -> Decode 4/1, Decode 3/1, Decode 2/1, Decode 1/1

== system speedgoat_test_SN5659_R2021b_IO682/IO682/Decode Channel 5 ==
  note: Because of the limited number of bits
      | that are encoded and sent by ARINC,
      | these values may differ from values
      | on the input side.
  In1 : Inport
  Decode 1 : speedgoatlib_IO682/Decode v2   parMode=Standard  parLabel=100  parDataType=[1]  parResolution=[1024]  parSyncMask=hex2dec('0x0')  parSyncValue=hex2dec('0x0')  parCustomDataType=Raw  parDataLSB=9  parDataMSB=31  parBitPosition=[9, 31]  parScaleBNR=1  parExponent=8  parMantissa=14  parTimeTags=off  parHoldLastVal=on  parStatus=off
      settings: SourceProductName=Simulink Real-Time: Speedgoat I/O Blockset
  Decode 3 : speedgoatlib_IO682/Decode v2   parMode=Standard  parLabel=102  parDataType=[1]  parResolution=[65536]  parSyncMask=hex2dec('0x0')  parSyncValue=hex2dec('0x0')  parCustomDataType=Raw  parDataLSB=9  parDataMSB=31  parBitPosition=[9, 31]  parScaleBNR=1  parExponent=8  parMantissa=14  parTimeTags=off  parHoldLastVal=on  parStatus=off
      settings: SourceProductName=Simulink Real-Time: Speedgoat I/O Blockset
  Decode 4 : speedgoatlib_IO682/Decode v2   parMode=Standard  parLabel=103  parDataType=[1]  parResolution=[1024]  parSyncMask=hex2dec('0x0')  parSyncValue=hex2dec('0x0')  parCustomDataType=Raw  parDataLSB=9  parDataMSB=31  parBitPosition=[9, 31]  parScaleBNR=1  parExponent=8  parMantissa=14  parTimeTags=off  parHoldLastVal=on  parStatus=off
      settings: SourceProductName=Simulink Real-Time: Speedgoat I/O Blockset
  Decode 5 : speedgoatlib_IO682/Decode v2   parMode=Standard  parLabel=101  parDataType=[2]  parResolution=[.1]  parSyncMask=hex2dec('0x0')  parSyncValue=hex2dec('0x0')  parCustomDataType=Raw  parDataLSB=9  parDataMSB=31  parBitPosition=[9, 31]  parScaleBNR=1  parExponent=8  parMantissa=14  parTimeTags=off  parHoldLastVal=on  parStatus=off
      settings: SourceProductName=Simulink Real-Time: Speedgoat I/O Blockset
  Mux : Mux
  Out1 : Outport
  wires:
  In1/1 -> Decode 3/1, Decode 4/1, Decode 5/1, Decode 1/1
  Mux/1 -> Out1/1
  Decode 5/1 -> Mux/2
  Decode 1/1 -> Mux/1
  Decode 3/1 -> Mux/3
  Decode 4/1 -> Mux/4

== system speedgoat_test_SN5659_R2021b_IO682/IO682/Decode Channel 6 ==
  In1 : Inport
  Decode 1 : speedgoatlib_IO682/Decode v2   parMode=Standard  parLabel=100  parDataType=[1]  parResolution=[1024]  parSyncMask=hex2dec('0x0')  parSyncValue=hex2dec('0x0')  parCustomDataType=Raw  parDataLSB=9  parDataMSB=31  parBitPosition=[9, 31]  parScaleBNR=1  parExponent=8  parMantissa=14  parTimeTags=off  parHoldLastVal=on  parStatus=off
      settings: SourceProductName=Simulink Real-Time: Speedgoat I/O Blockset
  Decode 2 : speedgoatlib_IO682/Decode v2   parMode=Standard  parLabel=101  parDataType=[2]  parResolution=[.1]  parSyncMask=hex2dec('0x0')  parSyncValue=hex2dec('0x0')  parCustomDataType=Raw  parDataLSB=9  parDataMSB=31  parBitPosition=[9, 31]  parScaleBNR=1  parExponent=8  parMantissa=14  parTimeTags=off  parHoldLastVal=on  parStatus=off
      settings: SourceProductName=Simulink Real-Time: Speedgoat I/O Blockset
  Decode 3 : speedgoatlib_IO682/Decode v2   parMode=Standard  parLabel=102  parDataType=[1]  parResolution=[65536]  parSyncMask=hex2dec('0x0')  parSyncValue=hex2dec('0x0')  parCustomDataType=Raw  parDataLSB=9  parDataMSB=31  parBitPosition=[9, 31]  parScaleBNR=1  parExponent=8  parMantissa=14  parTimeTags=off  parHoldLastVal=on  parStatus=off
      settings: SourceProductName=Simulink Real-Time: Speedgoat I/O Blockset
  Decode 4 : speedgoatlib_IO682/Decode v2   parMode=Standard  parLabel=103  parDataType=[1]  parResolution=[1024]  parSyncMask=hex2dec('0x0')  parSyncValue=hex2dec('0x0')  parCustomDataType=Raw  parDataLSB=9  parDataMSB=31  parBitPosition=[9, 31]  parScaleBNR=1  parExponent=8  parMantissa=14  parTimeTags=off  parHoldLastVal=on  parStatus=off
      settings: SourceProductName=Simulink Real-Time: Speedgoat I/O Blockset
  Mux : Mux
  Out1 : Outport
  wires:
  Decode 1/1 -> Mux/1
  In1/1 -> Decode 4/1, Decode 3/1, Decode 2/1, Decode 1/1
  Mux/1 -> Out1/1
  Decode 4/1 -> Mux/4
  Decode 3/1 -> Mux/3
  Decode 2/1 -> Mux/2

== system speedgoat_test_SN5659_R2021b_IO682/IO682/Decode Channel 7 ==
  In1 : Inport
  Decode 1 : speedgoatlib_IO682/Decode v2   parMode=Standard  parLabel=100  parDataType=[1]  parResolution=[1024]  parSyncMask=hex2dec('0x0')  parSyncValue=hex2dec('0x0')  parCustomDataType=Raw  parDataLSB=9  parDataMSB=31  parBitPosition=[9, 31]  parScaleBNR=1  parExponent=8  parMantissa=14  parTimeTags=off  parHoldLastVal=on  parStatus=off
      settings: SourceProductName=Simulink Real-Time: Speedgoat I/O Blockset
  Decode 2 : speedgoatlib_IO682/Decode v2   parMode=Standard  parLabel=101  parDataType=[2]  parResolution=[.1]  parSyncMask=hex2dec('0x0')  parSyncValue=hex2dec('0x0')  parCustomDataType=Raw  parDataLSB=9  parDataMSB=31  parBitPosition=[9, 31]  parScaleBNR=1  parExponent=8  parMantissa=14  parTimeTags=off  parHoldLastVal=on  parStatus=off
      settings: SourceProductName=Simulink Real-Time: Speedgoat I/O Blockset
  Decode 3 : speedgoatlib_IO682/Decode v2   parMode=Standard  parLabel=102  parDataType=[1]  parResolution=[65536]  parSyncMask=hex2dec('0x0')  parSyncValue=hex2dec('0x0')  parCustomDataType=Raw  parDataLSB=9  parDataMSB=31  parBitPosition=[9, 31]  parScaleBNR=1  parExponent=8  parMantissa=14  parTimeTags=off  parHoldLastVal=on  parStatus=off
      settings: SourceProductName=Simulink Real-Time: Speedgoat I/O Blockset
  Decode 4 : speedgoatlib_IO682/Decode v2   parMode=Standard  parLabel=103  parDataType=[1]  parResolution=[1024]  parSyncMask=hex2dec('0x0')  parSyncValue=hex2dec('0x0')  parCustomDataType=Raw  parDataLSB=9  parDataMSB=31  parBitPosition=[9, 31]  parScaleBNR=1  parExponent=8  parMantissa=14  parTimeTags=off  parHoldLastVal=on  parStatus=off
      settings: SourceProductName=Simulink Real-Time: Speedgoat I/O Blockset
  Mux : Mux
  Out1 : Outport
  wires:
  Decode 1/1 -> Mux/1
  Decode 2/1 -> Mux/2
  Decode 4/1 -> Mux/4
  Decode 3/1 -> Mux/3
  Mux/1 -> Out1/1
  In1/1 -> Decode 4/1, Decode 3/1, Decode 2/1, Decode 1/1

== system speedgoat_test_SN5659_R2021b_IO682/IO682/Decode Channel 8 ==
  In1 : Inport
  Decode 1 : speedgoatlib_IO682/Decode v2   parMode=Standard  parLabel=100  parDataType=[1]  parResolution=[1024]  parSyncMask=hex2dec('0x0')  parSyncValue=hex2dec('0x0')  parCustomDataType=Raw  parDataLSB=9  parDataMSB=31  parBitPosition=[9, 31]  parScaleBNR=1  parExponent=8  parMantissa=14  parTimeTags=off  parHoldLastVal=on  parStatus=off
      settings: SourceProductName=Simulink Real-Time: Speedgoat I/O Blockset
  Decode 2 : speedgoatlib_IO682/Decode v2   parMode=Standard  parLabel=101  parDataType=[2]  parResolution=[.1]  parSyncMask=hex2dec('0x0')  parSyncValue=hex2dec('0x0')  parCustomDataType=Raw  parDataLSB=9  parDataMSB=31  parBitPosition=[9, 31]  parScaleBNR=1  parExponent=8  parMantissa=14  parTimeTags=off  parHoldLastVal=on  parStatus=off
      settings: SourceProductName=Simulink Real-Time: Speedgoat I/O Blockset
  Decode 3 : speedgoatlib_IO682/Decode v2   parMode=Standard  parLabel=102  parDataType=[1]  parResolution=[65536]  parSyncMask=hex2dec('0x0')  parSyncValue=hex2dec('0x0')  parCustomDataType=Raw  parDataLSB=9  parDataMSB=31  parBitPosition=[9, 31]  parScaleBNR=1  parExponent=8  parMantissa=14  parTimeTags=off  parHoldLastVal=on  parStatus=off
      settings: SourceProductName=Simulink Real-Time: Speedgoat I/O Blockset
  Decode 4 : speedgoatlib_IO682/Decode v2   parMode=Standard  parLabel=103  parDataType=[1]  parResolution=[1024]  parSyncMask=hex2dec('0x0')  parSyncValue=hex2dec('0x0')  parCustomDataType=Raw  parDataLSB=9  parDataMSB=31  parBitPosition=[9, 31]  parScaleBNR=1  parExponent=8  parMantissa=14  parTimeTags=off  parHoldLastVal=on  parStatus=off
      settings: SourceProductName=Simulink Real-Time: Speedgoat I/O Blockset
  Mux : Mux
  Out1 : Outport
  wires:
  Decode 1/1 -> Mux/1
  Decode 2/1 -> Mux/2
  Decode 4/1 -> Mux/4
  Decode 3/1 -> Mux/3
  Mux/1 -> Out1/1
  In1/1 -> Decode 4/1, Decode 3/1, Decode 2/1, Decode 1/1

== system speedgoat_test_SN5659_R2021b_IO682/IO682/Decode Channel 9 ==
  note: Because of the limited number of bits
      | that are encoded and sent by ARINC,
      | these values may differ from values
      | on the input side.
  In1 : Inport
  Decode 1 : speedgoatlib_IO682/Decode v2   parMode=Standard  parLabel=100  parDataType=[1]  parResolution=[1024]  parSyncMask=hex2dec('0x0')  parSyncValue=hex2dec('0x0')  parCustomDataType=Raw  parDataLSB=9  parDataMSB=31  parBitPosition=[9, 31]  parScaleBNR=1  parExponent=8  parMantissa=14  parTimeTags=off  parHoldLastVal=on  parStatus=off
      settings: SourceProductName=Simulink Real-Time: Speedgoat I/O Blockset
  Decode 3 : speedgoatlib_IO682/Decode v2   parMode=Standard  parLabel=102  parDataType=[1]  parResolution=[65536]  parSyncMask=hex2dec('0x0')  parSyncValue=hex2dec('0x0')  parCustomDataType=Raw  parDataLSB=9  parDataMSB=31  parBitPosition=[9, 31]  parScaleBNR=1  parExponent=8  parMantissa=14  parTimeTags=off  parHoldLastVal=on  parStatus=off
      settings: SourceProductName=Simulink Real-Time: Speedgoat I/O Blockset
  Decode 4 : speedgoatlib_IO682/Decode v2   parMode=Standard  parLabel=103  parDataType=[1]  parResolution=[1024]  parSyncMask=hex2dec('0x0')  parSyncValue=hex2dec('0x0')  parCustomDataType=Raw  parDataLSB=9  parDataMSB=31  parBitPosition=[9, 31]  parScaleBNR=1  parExponent=8  parMantissa=14  parTimeTags=off  parHoldLastVal=on  parStatus=off
      settings: SourceProductName=Simulink Real-Time: Speedgoat I/O Blockset
  Decode 5 : speedgoatlib_IO682/Decode v2   parMode=Standard  parLabel=101  parDataType=[2]  parResolution=[.1]  parSyncMask=hex2dec('0x0')  parSyncValue=hex2dec('0x0')  parCustomDataType=Raw  parDataLSB=9  parDataMSB=31  parBitPosition=[9, 31]  parScaleBNR=1  parExponent=8  parMantissa=14  parTimeTags=off  parHoldLastVal=on  parStatus=off
      settings: SourceProductName=Simulink Real-Time: Speedgoat I/O Blockset
  Mux : Mux
  Out1 : Outport
  wires:
  In1/1 -> Decode 3/1, Decode 4/1, Decode 5/1, Decode 1/1
  Mux/1 -> Out1/1
  Decode 5/1 -> Mux/2
  Decode 1/1 -> Mux/1
  Decode 3/1 -> Mux/3
  Decode 4/1 -> Mux/4
